simulink model "simulation"  (R2024a)
settings: Solver=FixedStepAuto  StartTime=0.0  StopTime=30  FixedStep=ts  RelTol=1e-3
values from neighbouring files (symbols this model uses):
  A = [A1; A2; A3; A4; A5; A6]    [setup.m]
  B = [0, 0 ... (first row only)    [setup.m]
  C = [0, 0, 1, 0, 0, 0 ... (first row only)    [setup.m]
  D = [0 0 ... (first row only)    [setup.m]
  Ig = 10*(m*l^2)/3    (= 6)    [setup.m]
  m = 5    [setup.m]
  ni_r = 1    [setup.m]
  ni_x = 1    [setup.m]
  ni_y = 6    [setup.m]
  ts = 0.05    [setup.m]
  u_eq = [m*g; 0]    [setup.m]
  w = [1,      1 ... (first row only)    [setup.m]
  z_eq = z_init    [setup.m]
  z_init = [0;0;0;0;0;0]    [setup.m]
libraries: slpidlib x3, simulink x2
settings Model: Creator=enead  LastModifiedBy=enead

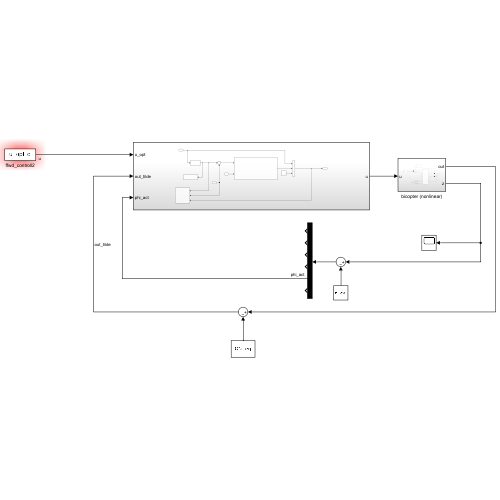
[thumbnail: Simulink's stored preview of the top-level diagram]
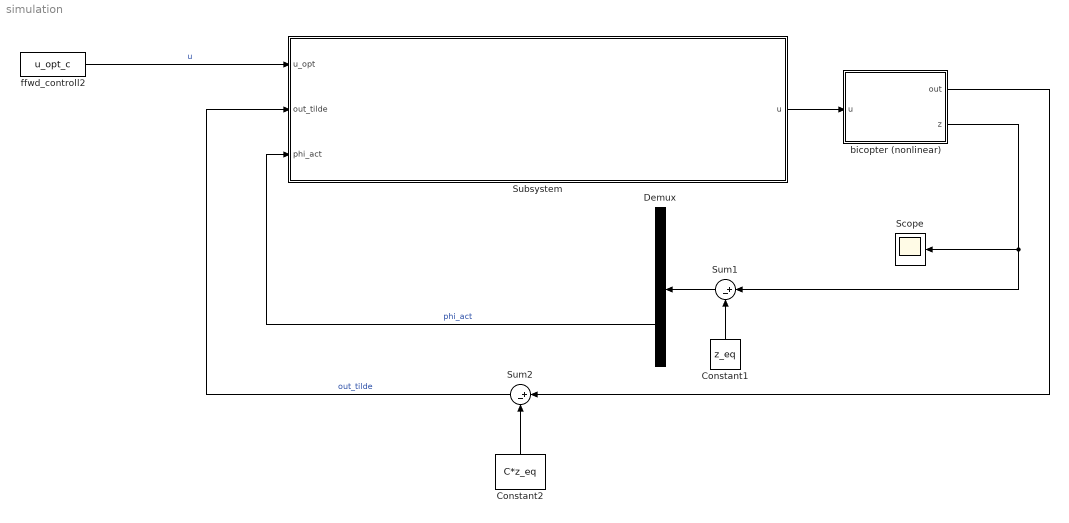
== system simulation ==
  Constant1 : Constant  Value=z_eq
  Constant2 : Constant  Value=C*z_eq
  Demux : Demux  Outputs=6
  Scope : Scope
  Subsystem : Subsystem
  Sum1 : Sum  Inputs=|+-
  Sum2 : Sum  Inputs=|+-
  bicopter (nonlinear) : Subsystem
  ffwd_controll2 : FromWorkspace  VariableName=u_opt_c  SampleTime=ts  OutputAfterFinalValue=Holding final value
  wires:
  Constant1/1 -> Sum1/2
  Sum1/1 -> Demux/1
  bicopter (nonlinear)/1(out) -> Sum2/1
  Constant2/1 -> Sum2/2
  Demux/5 -> Subsystem/3(phi_act)  "phi_act"
  Sum2/1 -> Subsystem/2(out_tilde)  "out_tilde"
  Subsystem/1(u) -> bicopter (nonlinear)/1(u)
  ffwd_controll2/1 -> Subsystem/1(u_opt)  "u"
  bicopter (nonlinear)/2(z) -> Sum1/1, Scope/1

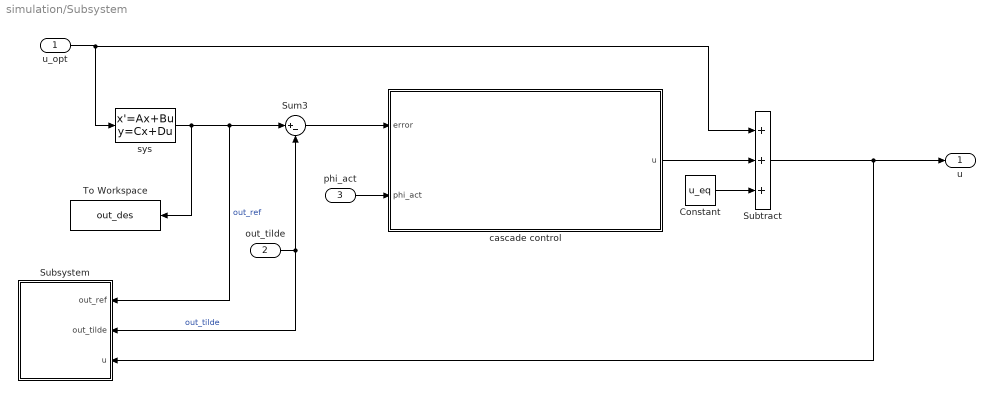
== system simulation/Subsystem ==
  u_opt : Inport
  out_tilde : Inport  Port=2
  phi_act : Inport  Port=3
  Constant : Constant  Value=u_eq
  Subsystem : Subsystem
  Subtract : Sum  Inputs=+++
  Sum3 : Sum  Inputs=|+-
  To Workspace : ToWorkspace  VariableName=out_des  SaveFormat=Timeseries  SampleTime=-1
  cascade control : Subsystem
  sys : StateSpace  A=A  B=B  C=C  D=D  InitialCondition=0
  u : Outport
  wires:
  sys/1 -> To Workspace/1, Sum3/1, Subsystem/1(out_ref)  "out_ref"
  cascade control/1(u) -> Subtract/2
  Sum3/1 -> cascade control/1(error)
  Constant/1 -> Subtract/3
  phi_act/1 -> cascade control/2(phi_act)
  u_opt/1 -> Subtract/1, sys/1
  Subtract/1 -> Subsystem/3(u), u/1
  out_tilde/1 -> Subsystem/2(out_tilde), Sum3/2  "out_tilde"

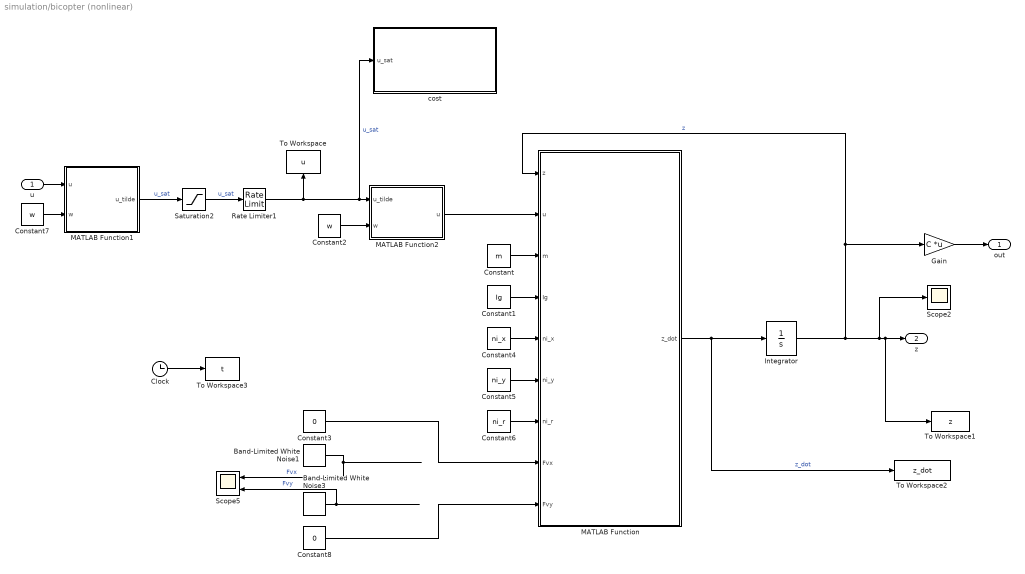
== system simulation/bicopter (nonlinear) ==
  u : Inport
  Band-Limited White Noise1 : simulink/Sources/Band-Limited White Noise  Cov=[7]  Ts=10  seed=[23341]
  Band-Limited White Noise3 : simulink/Sources/Band-Limited White Noise  Cov=[5]  Ts=15  seed=[23340]
  Clock : Clock
  Constant : Constant  Value=m
  Constant1 : Constant  Value=Ig
  Constant2 : Constant  Value=w
  Constant3 : Constant  Value=0
  Constant4 : Constant  Value=ni_x
  Constant5 : Constant  Value=ni_y  VectorParams1D=off
  Constant6 : Constant  Value=ni_r
  Constant7 : Constant  Value=w
  Constant8 : Constant  Value=0
  Gain : Gain  Gain=C  Multiplication=Matrix(K*u)
  Integrator : Integrator  InitialCondition=z_init
  MATLAB Function : MATLAB Function  TreatAsAtomicUnit=on
  MATLAB Function1 : MATLAB Function  TreatAsAtomicUnit=on
  MATLAB Function2 : MATLAB Function  TreatAsAtomicUnit=on
  Rate Limiter1 : RateLimiter  RisingSlewLimit=25  FallingSlewLimit=-25  SampleTimeMode=inherited
  Saturation2 : Saturate  UpperLimit=50  LowerLimit=0
  Scope2 : Scope
  Scope5 : Scope  NumInputPorts=2
  To Workspace : ToWorkspace  VariableName=u  SaveFormat=Timeseries  SampleTime=-1
  To Workspace1 : ToWorkspace  VariableName=z  SaveFormat=Timeseries  SampleTime=-1
  To Workspace2 : ToWorkspace  VariableName=z_dot  SaveFormat=Timeseries  SampleTime=-1
  To Workspace3 : ToWorkspace  VariableName=t  SaveFormat=Timeseries  SampleTime=-1
  cost : Subsystem
  out : Outport
  z : Outport  Port=2
  wires:
  Constant1/1 -> MATLAB Function/4(Ig)
  Integrator/1 -> Scope2/1, To Workspace1/1, z/1, Gain/1, MATLAB Function/1(z)  "z"
  Constant/1 -> MATLAB Function/3(m)
  MATLAB Function/1(z_dot) -> To Workspace2/1, Integrator/1  "z_dot"
  u/1 -> MATLAB Function1/1(u)
  Constant4/1 -> MATLAB Function/5(ni_x)
  Constant5/1 -> MATLAB Function/6(ni_y)
  Constant6/1 -> MATLAB Function/7(ni_r)
  MATLAB Function2/1(u) -> MATLAB Function/2(u)
  Constant2/1 -> MATLAB Function2/2(w)
  Constant7/1 -> MATLAB Function1/2(w)
  Clock/1 -> To Workspace3/1
  Gain/1 -> out/1
  MATLAB Function1/1(u_tilde) -> Saturation2/1  "u_sat"
  Saturation2/1 -> Rate Limiter1/1  "u_sat"
  Band-Limited White Noise3/1 -> Scope5/2  "Fvy"
  Band-Limited White Noise1/1 -> Scope5/1  "Fvx"
  Constant3/1 -> MATLAB Function/8(Fvx)
  Constant8/1 -> MATLAB Function/9(Fvy)
  Rate Limiter1/1 -> cost/1(u_sat), MATLAB Function2/1(u_tilde), To Workspace/1  "u_sat"

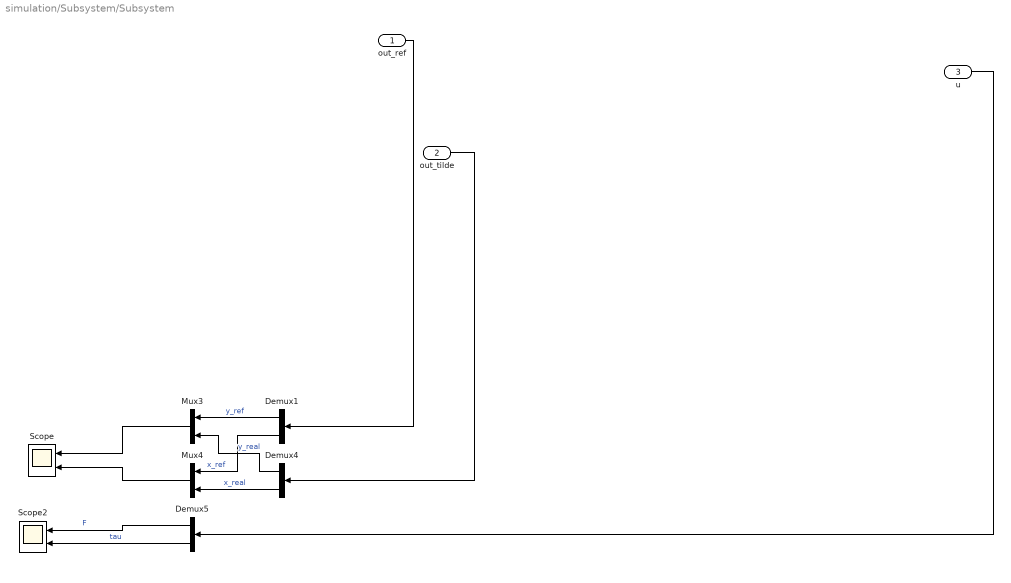
== system simulation/Subsystem/Subsystem ==
  out_ref : Inport
  out_tilde : Inport  Port=2
  u : Inport  Port=3
  Demux1 : Demux  Outputs=2
  Demux4 : Demux  Outputs=2
  Demux5 : Demux  Outputs=2
  Mux3 : Mux  Inputs=2
  Mux4 : Mux  Inputs=2
  Scope : Scope  NumInputPorts=2
  Scope2 : Scope  NumInputPorts=2
  wires:
  Mux3/1 -> Scope/1
  Demux1/2 -> Mux4/1  "x_ref"
  Demux5/1 -> Scope2/1  "F"
  Demux1/1 -> Mux3/1  "y_ref"
  Demux4/2 -> Mux4/2  "x_real"
  Mux4/1 -> Scope/2
  Demux5/2 -> Scope2/2  "tau"
  Demux4/1 -> Mux3/2  "y_real"
  u/1 -> Demux5/1
  out_ref/1 -> Demux1/1
  out_tilde/1 -> Demux4/1

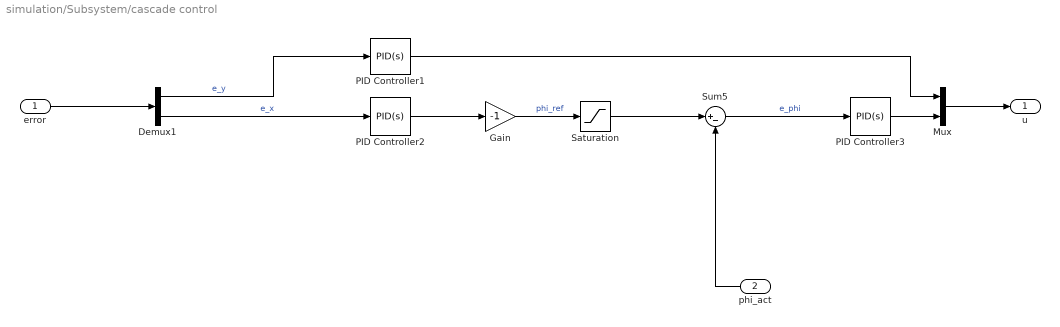
== system simulation/Subsystem/cascade control ==
  error : Inport
  phi_act : Inport  Port=2
  Demux1 : Demux  Outputs=2
  Gain : Gain  Gain=-1
  Mux : Mux  Inputs=2
  PID Controller1 : slpidlib/PID Controller  Controller=PID  Form=Parallel  TimeDomain=Continuous-time  UseExternalTs=off  SampleTime=-1  IntegratorMethod=Forward Euler  FilterMethod=Forward Euler  ControllerParametersSource=internal  P=12  I=0  UseKiTs=off  D=13  UseExternalDerivativeSource=off  N=30  UseFilter=on  TunerSelectOption=Transfer Function Based (PID Tuner App)  InitialConditionSource=internal  InitialConditionForIntegrator=0  InitialConditionForFilter=0  DifferentiatorICPrevScaledInput=0  ExternalReset=none  TrackingMode=off  Kt=1  LimitOutput=off  SatLimitsSource=internal  UpperSaturationLimit=inf  LowerSaturationLimit=-inf  LinearizeAsGain=on  AntiWindupMode=none  Kb=1  LimitIntegrator=off  UpperIntegratorSaturationLimit=inf  LowerIntegratorSaturationLimit=-inf  POutMin=[]  POutMax=[]  IOutMin=[]  IOutMax=[]  DOutMin=[]  DOutMax=[]  NOutMin=[]  NOutMax=[]  SumOutMin=[]  SumOutMax=[]  SaturationOutMin=[]  SaturationOutMax=[]  PParamMin=[]  PParamMax=[]  IParamMin=[]  IParamMax=[]  DParamMin=[]  DParamMax=[]  NParamMin=[]  NParamMax=[]  KbParamMin=[]  KbParamMax=[]  KtParamMin=[]  KtParamMax=[]  KbOutMin=[]  KbOutMax=[]  KtOutMin=[]  KtOutMax=[]  IntegratorOutMin=[]  IntegratorOutMax=[]  FilterOutMin=[]  FilterOutMax=[]  SumI1OutMin=[]  SumI1OutMax=[]  SumI2OutMin=[]  SumI2OutMax=[]  SumI3OutMin=[]  SumI3OutMax=[]  SumI4OutMin=[]  SumI4OutMax=[]  SumDOutMin=[]  SumDOutMax=[]  DifferentiatorOutMin=[]  DifferentiatorOutMax=[]  FilterDiffOutCoefMin=[]  FilterDiffOutCoefMax=[]  ReciprocalOutMin=[]  ReciprocalOutMax=[]  SumDenOutMin=[]  SumDenOutMax=[]  SumNumOutMin=[]  SumNumOutMax=[]  DivideOutMin=[]  DivideOutMax=[]  UdiffTsProdOutMin=[]  UdiffTsProdOutMax=[]  NTsProdOutMin=[]  NTsProdOutMax=[]  UintegralTsProdOutMin=[]  UintegralTsProdOutMax=[]  UngainTsProdOutMin=[]  UngainTsProdOutMax=[]  ClampingZeroOutDataTypeStr=Inherit: Inherit via back propagation  ClampingZeroOutMin=[]  ClampingZeroOutMax=[]  FilterDenConstantOutDataTypeStr=Inherit: Inherit via back propagation  FilterDenConstantOutMin=[]  FilterDenConstantOutMax=[]  PCopyOutDataTypeStr=Inherit: Inherit via back propagation  PCopyOutMin=[]  PCopyOutMax=[]  NCopyOutDataTypeStr=Inherit: Inherit via back propagation  NCopyOutMin=[]  NCopyOutMax=[]  IntegratorContinuousStateAttributes=''  IntegratorStateMustResolveToSignalObject=off  IntegratorRTWStateStorageClass=Auto  FilterContinuousStateAttributes=''  FilterStateMustResolveToSignalObject=off  FilterRTWStateStorageClass=Auto  ParallelPVariant=InternalParameters  IdealPVariant=Disabled  IVariant=InternalParameters  DVariant=InternalParameters  IntegratorVariant=Continuous  SatVariant=Disabled  AWVariant=Passthrough  PCopyVariant=Disabled  TRVariant=Disabled  FdbkBlocksVariant=Forward  IdealPFdbkVariant=Disabled  SatFdbkVariant=Disabled  DerivativeFilterVariant=ContFilter  NVariant=InternalParameters  NCopyVariant=Disabled  FilterICVariant=InternalICsFilter  IntegratorICVariant=InternalICs  ExternalResetVariant=Disabled  TRSumVariant=Passthrough  SumFdbkVariant=Disabled  SumVariant=Sum_PID  TsampFilterVariant=InternalTs  TsampNgainVariant=Passthrough  TsampIntegralVariant=Disabled_SignalSpec  ExternalSaturationOutDataTypeStr=Inherit: Same as second input  DerivativeSourceVariant=ErrorSignal
  PID Controller2 : slpidlib/PID Controller  Controller=PID  Form=Parallel  TimeDomain=Continuous-time  UseExternalTs=off  SampleTime=-1  IntegratorMethod=Forward Euler  FilterMethod=Forward Euler  ControllerParametersSource=internal  P=0.09  I=0  UseKiTs=off  D=0.17  UseExternalDerivativeSource=off  N=14  UseFilter=on  TunerSelectOption=Transfer Function Based (PID Tuner App)  InitialConditionSource=internal  InitialConditionForIntegrator=0  InitialConditionForFilter=0  DifferentiatorICPrevScaledInput=0  ExternalReset=none  TrackingMode=off  Kt=1  LimitOutput=off  SatLimitsSource=internal  UpperSaturationLimit=inf  LowerSaturationLimit=-inf  LinearizeAsGain=on  AntiWindupMode=none  Kb=1  LimitIntegrator=off  UpperIntegratorSaturationLimit=inf  LowerIntegratorSaturationLimit=-inf  POutMin=[]  POutMax=[]  IOutMin=[]  IOutMax=[]  DOutMin=[]  DOutMax=[]  NOutMin=[]  NOutMax=[]  SumOutMin=[]  SumOutMax=[]  SaturationOutMin=[]  SaturationOutMax=[]  PParamMin=[]  PParamMax=[]  IParamMin=[]  IParamMax=[]  DParamMin=[]  DParamMax=[]  NParamMin=[]  NParamMax=[]  KbParamMin=[]  KbParamMax=[]  KtParamMin=[]  KtParamMax=[]  KbOutMin=[]  KbOutMax=[]  KtOutMin=[]  KtOutMax=[]  IntegratorOutMin=[]  IntegratorOutMax=[]  FilterOutMin=[]  FilterOutMax=[]  SumI1OutMin=[]  SumI1OutMax=[]  SumI2OutMin=[]  SumI2OutMax=[]  SumI3OutMin=[]  SumI3OutMax=[]  SumI4OutMin=[]  SumI4OutMax=[]  SumDOutMin=[]  SumDOutMax=[]  DifferentiatorOutMin=[]  DifferentiatorOutMax=[]  FilterDiffOutCoefMin=[]  FilterDiffOutCoefMax=[]  ReciprocalOutMin=[]  ReciprocalOutMax=[]  SumDenOutMin=[]  SumDenOutMax=[]  SumNumOutMin=[]  SumNumOutMax=[]  DivideOutMin=[]  DivideOutMax=[]  UdiffTsProdOutMin=[]  UdiffTsProdOutMax=[]  NTsProdOutMin=[]  NTsProdOutMax=[]  UintegralTsProdOutMin=[]  UintegralTsProdOutMax=[]  UngainTsProdOutMin=[]  UngainTsProdOutMax=[]  ClampingZeroOutDataTypeStr=Inherit: Inherit via back propagation  ClampingZeroOutMin=[]  ClampingZeroOutMax=[]  FilterDenConstantOutDataTypeStr=Inherit: Inherit via back propagation  FilterDenConstantOutMin=[]  FilterDenConstantOutMax=[]  PCopyOutDataTypeStr=Inherit: Inherit via back propagation  PCopyOutMin=[]  PCopyOutMax=[]  NCopyOutDataTypeStr=Inherit: Inherit via back propagation  NCopyOutMin=[]  NCopyOutMax=[]  IntegratorContinuousStateAttributes=''  IntegratorStateMustResolveToSignalObject=off  IntegratorRTWStateStorageClass=Auto  FilterContinuousStateAttributes=''  FilterStateMustResolveToSignalObject=off  FilterRTWStateStorageClass=Auto  ParallelPVariant=InternalParameters  IdealPVariant=Disabled  IVariant=InternalParameters  DVariant=InternalParameters  IntegratorVariant=Continuous  SatVariant=Disabled  AWVariant=Passthrough  PCopyVariant=Disabled  TRVariant=Disabled  FdbkBlocksVariant=Forward  IdealPFdbkVariant=Disabled  SatFdbkVariant=Disabled  DerivativeFilterVariant=ContFilter  NVariant=InternalParameters  NCopyVariant=Disabled  FilterICVariant=InternalICsFilter  IntegratorICVariant=InternalICs  ExternalResetVariant=Disabled  TRSumVariant=Passthrough  SumFdbkVariant=Disabled  SumVariant=Sum_PID  TsampFilterVariant=InternalTs  TsampNgainVariant=Passthrough  TsampIntegralVariant=Disabled_SignalSpec  ExternalSaturationOutDataTypeStr=Inherit: Same as second input  DerivativeSourceVariant=ErrorSignal
  PID Controller3 : slpidlib/PID Controller  Controller=PID  Form=Parallel  TimeDomain=Continuous-time  UseExternalTs=off  SampleTime=-1  IntegratorMethod=Forward Euler  FilterMethod=Forward Euler  ControllerParametersSource=internal  P=5  I=0  UseKiTs=off  D=28  UseExternalDerivativeSource=off  N=10  UseFilter=on  TunerSelectOption=Transfer Function Based (PID Tuner App)  InitialConditionSource=internal  InitialConditionForIntegrator=0  InitialConditionForFilter=0  DifferentiatorICPrevScaledInput=0  ExternalReset=none  TrackingMode=off  Kt=1  LimitOutput=off  SatLimitsSource=internal  UpperSaturationLimit=inf  LowerSaturationLimit=-inf  LinearizeAsGain=on  AntiWindupMode=none  Kb=1  LimitIntegrator=off  UpperIntegratorSaturationLimit=inf  LowerIntegratorSaturationLimit=-inf  POutMin=[]  POutMax=[]  IOutMin=[]  IOutMax=[]  DOutMin=[]  DOutMax=[]  NOutMin=[]  NOutMax=[]  SumOutMin=[]  SumOutMax=[]  SaturationOutMin=[]  SaturationOutMax=[]  PParamMin=[]  PParamMax=[]  IParamMin=[]  IParamMax=[]  DParamMin=[]  DParamMax=[]  NParamMin=[]  NParamMax=[]  KbParamMin=[]  KbParamMax=[]  KtParamMin=[]  KtParamMax=[]  KbOutMin=[]  KbOutMax=[]  KtOutMin=[]  KtOutMax=[]  IntegratorOutMin=[]  IntegratorOutMax=[]  FilterOutMin=[]  FilterOutMax=[]  SumI1OutMin=[]  SumI1OutMax=[]  SumI2OutMin=[]  SumI2OutMax=[]  SumI3OutMin=[]  SumI3OutMax=[]  SumI4OutMin=[]  SumI4OutMax=[]  SumDOutMin=[]  SumDOutMax=[]  DifferentiatorOutMin=[]  DifferentiatorOutMax=[]  FilterDiffOutCoefMin=[]  FilterDiffOutCoefMax=[]  ReciprocalOutMin=[]  ReciprocalOutMax=[]  SumDenOutMin=[]  SumDenOutMax=[]  SumNumOutMin=[]  SumNumOutMax=[]  DivideOutMin=[]  DivideOutMax=[]  UdiffTsProdOutMin=[]  UdiffTsProdOutMax=[]  NTsProdOutMin=[]  NTsProdOutMax=[]  UintegralTsProdOutMin=[]  UintegralTsProdOutMax=[]  UngainTsProdOutMin=[]  UngainTsProdOutMax=[]  ClampingZeroOutDataTypeStr=Inherit: Inherit via back propagation  ClampingZeroOutMin=[]  ClampingZeroOutMax=[]  FilterDenConstantOutDataTypeStr=Inherit: Inherit via back propagation  FilterDenConstantOutMin=[]  FilterDenConstantOutMax=[]  PCopyOutDataTypeStr=Inherit: Inherit via back propagation  PCopyOutMin=[]  PCopyOutMax=[]  NCopyOutDataTypeStr=Inherit: Inherit via back propagation  NCopyOutMin=[]  NCopyOutMax=[]  IntegratorContinuousStateAttributes=''  IntegratorStateMustResolveToSignalObject=off  IntegratorRTWStateStorageClass=Auto  FilterContinuousStateAttributes=''  FilterStateMustResolveToSignalObject=off  FilterRTWStateStorageClass=Auto  ParallelPVariant=InternalParameters  IdealPVariant=Disabled  IVariant=InternalParameters  DVariant=InternalParameters  IntegratorVariant=Continuous  SatVariant=Disabled  AWVariant=Passthrough  PCopyVariant=Disabled  TRVariant=Disabled  FdbkBlocksVariant=Forward  IdealPFdbkVariant=Disabled  SatFdbkVariant=Disabled  DerivativeFilterVariant=ContFilter  NVariant=InternalParameters  NCopyVariant=Disabled  FilterICVariant=InternalICsFilter  IntegratorICVariant=InternalICs  ExternalResetVariant=Disabled  TRSumVariant=Passthrough  SumFdbkVariant=Disabled  SumVariant=Sum_PID  TsampFilterVariant=InternalTs  TsampNgainVariant=Passthrough  TsampIntegralVariant=Disabled_SignalSpec  ExternalSaturationOutDataTypeStr=Inherit: Same as second input  DerivativeSourceVariant=ErrorSignal
  Saturation : Saturate  UpperLimit=2  LowerLimit=-2
  Sum5 : Sum  Inputs=|+-
  u : Outport
  wires:
  Saturation/1 -> Sum5/1
  PID Controller2/1 -> Gain/1
  Demux1/2 -> PID Controller2/1  "e_x"
  PID Controller3/1 -> Mux/2
  Sum5/1 -> PID Controller3/1  "e_phi"
  PID Controller1/1 -> Mux/1
  Demux1/1 -> PID Controller1/1  "e_y"
  Gain/1 -> Saturation/1  "phi_ref"
  phi_act/1 -> Sum5/2
  error/1 -> Demux1/1
  Mux/1 -> u/1

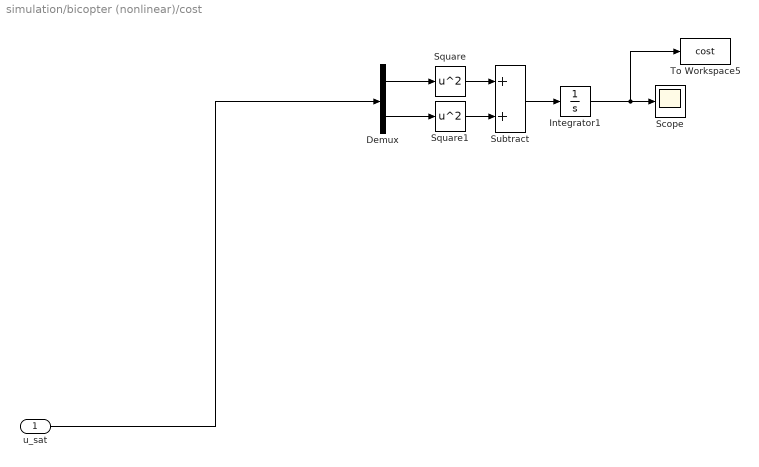
== system simulation/bicopter (nonlinear)/cost ==
  u_sat : Inport
  Demux : Demux  Outputs=2
  Integrator1 : Integrator
  Scope : Scope
  Square : Math  Operator=square
  Square1 : Math  Operator=square
  Subtract : Sum
  To Workspace5 : ToWorkspace  VariableName=cost  SaveFormat=Timeseries  SampleTime=-1
  wires:
  Square1/1 -> Subtract/2
  Subtract/1 -> Integrator1/1
  u_sat/1 -> Demux/1
  Square/1 -> Subtract/1
  Demux/1 -> Square/1
  Integrator1/1 -> To Workspace5/1, Scope/1
  Demux/2 -> Square1/1

== matlab function simulation/bicopter (nonlinear)/MATLAB Function ==
  data: z input; u input; z_dot output; m input; Ig input; ni_x input; ni_y input; ni_r input; Fvx input; Fvy input
function z_dot = drone_nonlinear_evol(z, u, m, Ig, ni_x, ni_y, ni_r, Fvx, Fvy)

    g = 9.81;

    x = z(1);
    x_dot = z(2);
    y = z(3);
    y_dot = z(4);
    phi = z(5);
    phi_dot = z(6);

    F = u(1);
    tau = u(2);

    z_dot1 = x_dot;
    z_dot2 = - F/m * sin(phi) - ni_x*x_dot*sin(phi)/m - Fvx/m;
    z_dot3 = y_dot;
    z_dot4 = F/m * cos(phi) - g  - ni_y*y_dot*cos(phi)/m - Fvy/m;
    z_dot5 = phi_dot;
    z_dot6 = tau/Ig - ni_r*phi_dot/Ig;

    z_dot = [z_dot1; z_dot2; z_dot3; z_dot4; z_dot5; z_dot6];

== matlab function simulation/bicopter (nonlinear)/MATLAB Function1 ==
  data: u input; u_tilde output; w input
function u_tilde = tilding(u, w)

    u_tilde = w\u;

== matlab function simulation/bicopter (nonlinear)/MATLAB Function2 ==
  data: u_tilde input; u output; w input
function u = detilding(u_tilde, w)

    u = w*u_tilde;
